simulink model "sampleModel7288_pp_1_1"  (R2018a)
settings: Solver=VariableStepAuto  StartTime=0.0  StopTime=10.0  RelTol=1e-3
undefined symbols (not defined in the file): DiscIntNeverNeededParam, sigbuilder_block
libraries: simulink x497
(part 1 of 10)
settings Model: Creator=cyfuzz  LastModifiedBy=shafiul
settings CodeAppCC: StateflowObjectComments=on

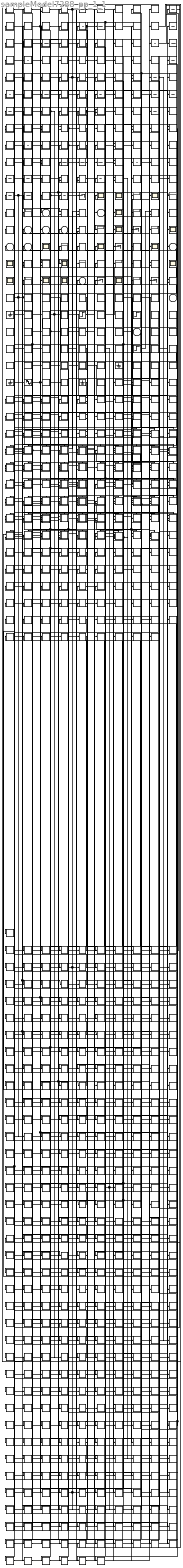
== system sampleModel7288_pp_1_1 ==
  cfblk180 : Inport
  cfblk198 : Inport  Port=2
  cfblk{1,9,50,54..55,58,83,85,88} (9 alike) : simulink/Discrete/Difference  ICPrevInput=0.0  OutMin=[]  OutMax=[]  OutDataTypeStr=double  OutputDataTypeScalingMode=double  OutDataType=fixdt(1, 16)  OutScaling=2^-10  DoSatur=off
  cfblk{10,20,40,56,59..60,102,106,111,114} (10 alike) : DiscreteIntegrator  OutDataTypeStr=double  ICPrevOutput=DiscIntNeverNeededParam  ICPrevScaledInput=DiscIntNeverNeededParam
  cfblk{28,77,89,100} (4 alike) : simulink/Discrete/Transfer Fcn Lead or Lag  PoleZ=0.95  ZeroZ=0.75  ICPrevOutput=0.0  ICPrevInput=0.0  DoSatur=off
      settings: SourceProductName=Simulink  SourceProductBaseCode=SL
  cfblk{5,16,49,53,61,69,96,101} (8 alike) : DiscreteTransferFcn  SampleTime=1
  cfblk{12,39,45,103} (4 alike) : simulink/Discrete/Transfer Fcn Real Zero  ZeroZ=0.75  ICPrevInput=0.0  DoSatur=off
      settings: SourceProductName=Simulink  SourceProductBaseCode=SL
  cfblk{71,80,92,97,104..105} (6 alike) : simulink/Continuous/PID Controller (2DOF)  Controller=PID  TimeDomain=Discrete-time  SampleTime=1  IntegratorMethod=Forward Euler  FilterMethod=Forward Euler  Form=Parallel  UseFilter=on  ControllerParametersSource=internal  P=1  I=1  D=0  N=100  b=1  c=1  InitialConditionSource=internal  InitialConditionForIntegrator=0  InitialConditionForFilter=0  ExternalReset=none  LimitOutput=off  UpperSaturationLimit=inf  LowerSaturationLimit=-inf  LinearizeAsGain=off  AntiWindupMode=none  Kb=1  TrackingMode=off  Kt=1  PParamMin=[]  PParamMax=[]  IParamMin=[]  IParamMax=[]  DParamMin=[]  DParamMax=[]  NParamMin=[]  NParamMax=[]  bParamMin=[]  bParamMax=[]  cParamMin=[]  cParamMax=[]  KbParamMin=[]  KbParamMax=[]  KtParamMin=[]  KtParamMax=[]  POutMin=[]  POutMax=[]  IOutMin=[]  IOutMax=[]  DOutMin=[]  DOutMax=[]  NOutMin=[]  NOutMax=[]  bOutMin=[]  bOutMax=[]  cOutMin=[]  cOutMax=[]  KbOutMin=[]  KbOutMax=[]  KtOutMin=[]  KtOutMax=[]  IntegratorOutMin=[]  IntegratorOutMax=[]  FilterOutMin=[]  FilterOutMax=[]  SumOutMin=[]  SumOutMax=[]  Sum1OutMin=[]  Sum1OutMax=[]  Sum2OutMin=[]  Sum2OutMax=[]  Sum3OutMin=[]  Sum3OutMax=[]  SumI1OutMin=[]  SumI1OutMax=[]  SumI2OutMin=[]  SumI2OutMax=[]  SumI3OutMin=[]  SumI3OutMax=[]  SumDOutMin=[]  SumDOutMax=[]  SaturationOutMin=[]  SaturationOutMax=[]  IntegratorContinuousStateAttributes=''  IntegratorStateMustResolveToSignalObject=off  IntegratorRTWStateStorageClass=Auto  FilterContinuousStateAttributes=''  FilterStateMustResolveToSignalObject=off  FilterRTWStateStorageClass=Auto  DifferentiatorICPrevScaledInput=0  DifferentiatorOutMin=[]  DifferentiatorOutMax=[]  FilterDiffOutCoefMin=[]  FilterDiffOutCoefMax=[]  SumDenOutMin=[]  SumDenOutMax=[]  SumNumOutMin=[]  SumNumOutMax=[]  ReciprocalOutMin=[]  ReciprocalOutMax=[]  DivideOutMin=[]  DivideOutMax=[]  TunerSelectOption=Transfer Function Based (PID Tuner App)
  cfblk{3,22,48,72..74,87,107} (8 alike) : Delay  DelayLengthSource=Input port  SampleTime=1
      settings: InputPortMap=u0,p1
  cfblk{43,65,76,84,91,108..109} (7 alike) : DiscreteZeroPole  Poles=[0 0.5]  Gain=1
  cfblk{7,11,44,52,63,90} (6 alike) : simulink/Discrete/Transfer Fcn First Order  PoleZ=0.95  ICPrevOutput=0.0  DoSatur=off
      settings: SourceProductName=Simulink
  cfblk{18,26,34..35,46,57,68,81,86,99,110} (11 alike) : simulink/Continuous/PID Controller  Controller=PID  TimeDomain=Discrete-time  SampleTime=1  IntegratorMethod=Forward Euler  FilterMethod=Forward Euler  Form=Parallel  UseFilter=on  ControllerParametersSource=internal  P=1  I=1  D=0  N=100  InitialConditionSource=internal  InitialConditionForIntegrator=0  InitialConditionForFilter=0  ExternalReset=none  LimitOutput=off  UpperSaturationLimit=inf  LowerSaturationLimit=-inf  LinearizeAsGain=off  AntiWindupMode=none  Kb=1  TrackingMode=off  Kt=1  PParamMin=[]  PParamMax=[]  IParamMin=[]  IParamMax=[]  DParamMin=[]  DParamMax=[]  NParamMin=[]  NParamMax=[]  KbParamMin=[]  KbParamMax=[]  KtParamMin=[]  KtParamMax=[]  POutMin=[]  POutMax=[]  IOutMin=[]  IOutMax=[]  DOutMin=[]  DOutMax=[]  NOutMin=[]  NOutMax=[]  KbOutMin=[]  KbOutMax=[]  KtOutMin=[]  KtOutMax=[]  IntegratorOutMin=[]  IntegratorOutMax=[]  FilterOutMin=[]  FilterOutMax=[]  SumOutMin=[]  SumOutMax=[]  SumI1OutMin=[]  SumI1OutMax=[]  SumI2OutMin=[]  SumI2OutMax=[]  SumI3OutMin=[]  SumI3OutMax=[]  SumDOutMin=[]  SumDOutMax=[]  SaturationOutMin=[]  SaturationOutMax=[]  IntegratorContinuousStateAttributes=''  IntegratorStateMustResolveToSignalObject=off  IntegratorRTWStateStorageClass=Auto  FilterContinuousStateAttributes=''  FilterStateMustResolveToSignalObject=off  FilterRTWStateStorageClass=Auto  DifferentiatorICPrevScaledInput=0  DifferentiatorOutMin=[]  DifferentiatorOutMax=[]  FilterDiffOutCoefMin=[]  FilterDiffOutCoefMax=[]  SumDenOutMin=[]  SumDenOutMax=[]  SumNumOutMin=[]  SumNumOutMax=[]  ReciprocalOutMin=[]  ReciprocalOutMax=[]  DivideOutMin=[]  DivideOutMax=[]  TunerSelectOption=Transfer Function Based (PID Tuner App)
  cfblk{6,23,30,94..95,112} (6 alike) : DiscreteFilter  SampleTime=1
  cfblk{8,19,24..25,31,37..38,62,64,67,113,320..375} (67 alike) : Delay  SampleTime=1
  cfblk{115,138,147,166,169} (5 alike) : Terminator
  cfblk{116..117,119,127,137,140,143,146,149,151,154,160..161,163..164,167} (16 alike) : Scope
      cfblk117 settings: Floating=on
      cfblk143 settings: Floating=on
      cfblk151 settings: Floating=on
      cfblk160 settings: Floating=on
      cfblk161 settings: Floating=on
      cfblk164 settings: Floating=on
      cfblk167 settings: Floating=on
  cfblk{118,120,122,128,136,139,144,155,157,162,168} (11 alike) : Display
  cfblk121 : ToWorkspace  VariableName=ajgaihg  SaveFormat=Timeseries  SampleTime=-1
  cfblk{124..125,129,135,152..153,159,170} (8 alike) : simulink/Sinks/XY Graph  xmin=-1  xmax=1  ymin=-1  ymax=1  st=-1
  cfblk{2,13..14,21,27,36,41..42,47,75} (10 alike) : simulink/Discrete/Tapped Delay  vinit=0.0  samptime=-1  NumDelays=1  DelayOrder=Oldest  includeCurrent=off
  cfblk130 : ToWorkspace  VariableName=uwfehsf  SaveFormat=Timeseries  SampleTime=-1
  cfblk131 : ToWorkspace  VariableName=zgsnsfd  SaveFormat=Timeseries  SampleTime=-1
  cfblk145 : ToWorkspace  VariableName=qxglayd  SaveFormat=Timeseries  SampleTime=-1
  cfblk148 : ToWorkspace  VariableName=ajdkbiq  SaveFormat=Timeseries  SampleTime=-1
  cfblk{15,29,32,51,82,98} (6 alike) : UnitDelay
  cfblk156 : ToWorkspace  VariableName=zvxkfyp  SaveFormat=Timeseries  SampleTime=-1
  cfblk158 : ToWorkspace  VariableName=xydmkth  SaveFormat=Timeseries  SampleTime=-1
  cfblk{4,17,33,70,79} (5 alike) : DiscreteStateSpace
  cfblk171 : simulink/Sources/Band-Limited White Noise  Cov=[0.1]  Ts=0.1  seed=[23341]
  cfblk{172,174,182,192,196,211,216} (7 alike) : simulink/Sources/Counter Limited  uplimit=7  tsamp=1
  cfblk173 : simulink/Sources/Band-Limited White Noise  Cov=[0.1]  Ts=0.1  seed=[23341]
  cfblk175 : DigitalClock
  cfblk176 : simulink/Sources/Counter Free-Running  NumBits=16  tsamp=1
  cfblk{177,179,191,197,204,207,226} (7 alike) : SignalGenerator  Units=rad/sec
  cfblk178 : simulink/Sources/Chirp Signal  f1=0.1  T=100  f2=1
  cfblk{181,217,221,225} (4 alike) : Ground
  cfblk183 : simulink/Sources/Ramp  slope=1  start=0  InitialOutput=0
  cfblk184 : simulink/Sources/Chirp Signal  f1=0.1  T=100  f2=1
  cfblk185 : Step  After=67  SampleTime=0
  cfblk{186,210,220,224} (4 alike) : simulink/Sources/Repeating Sequence  rep_seq_t=[0 2]  rep_seq_y=[0 2]
  cfblk{187,189..190,199,205,223} (6 alike) : DiscretePulseGenerator  PulseType=Time based  Period=10  PulseWidth=5
  cfblk188 : Step  After=98  SampleTime=0
  cfblk{193,206,212,219} (4 alike) : simulink/Sources/Repeating Sequence Interpolated  OutValues=[3 1 4 2 1].'  TimeValues=[0 0.1 0.5 0.6 1].'  LookUpMeth=Interpolation-Use End Values  tsamp=0.01  OutMin=[]  OutMax=[]  OutDataTypeStr=double  OutputDataTypeScalingMode=double  OutDataType=fixdt(0,8)  OutScaling=2^-10
  cfblk194 : UniformRandomNumber  SampleTime=0.1
  cfblk195 : UniformRandomNumber  SampleTime=0.1
  cfblk200 : Subsystem  Tag=STV Subsys  LoadFcn=sigbuilder_block('load');  StartFcn=sigbuilder_block('start');  StopFcn=sigbuilder_block('stop');  ClipboardFcn=sigbuilder_block('clipboard');  mask(Sigbuilder block){tuvar=[0:10]}
      mask help: Simulink:masks:SigbuilderBlock_MD
      mask init:
      | if ~strcmp(get_param(bdroot(gcbh),'SimulationStatus'),'stopped') tuvar = sigbuilder_block('maskInit'); end
      settings: CopyFcn=sigbuilder_block('copy');  DeleteFcn=sigbuilder_block('delete');  ModelCloseFcn=sigbuilder_block('modelClose');  PreSaveFcn=sigbuilder_block('preSave');  PauseFcn=sigbuilder_block('pause');  ContinueFcn=sigbuilder_block('continue');  NameChangeFcn=sigbuilder_block('namechange');  OpenFcn=sigbuilder_block('open',[437.6 199.2 550.4 400 ]);  CloseFcn=sigbuilder_block('close');
      mask Display: plot(0, 0, 100, 100,[2, 2, 32, 32, 2], [68, 8, 8, 68, 68],[32, 2], [38, 38], [32, 19, 2],[53, 60, 44], [32, 17, 17, 2],[16, 16, 31, 31]);txt = getActiveGroup(gcbh);text(2, 100, txt,'verticalAlignment', 'top');
  cfblk201 : simulink/Sources/Ramp  slope=1  start=0  InitialOutput=0
  cfblk202 : simulink/Sources/Repeating Sequence Stair  OutValues=[3 1 4 2 1].'  tsamp=1  OutMin=[]  OutMax=[]  OutDataTypeStr=double  OutputDataTypeScalingMode=double  OutDataType=fixdt(0,8)  ConRadixGroup=Best Precision: Vector-wise  OutScaling=2^-12
  cfblk203 : simulink/Sources/Repeating Sequence Stair  OutValues=[3 1 4 2 1].'  tsamp=1  OutMin=[]  OutMax=[]  OutDataTypeStr=double  OutputDataTypeScalingMode=double  OutDataType=fixdt(0,8)  ConRadixGroup=Best Precision: Vector-wise  OutScaling=2^-12
  cfblk208 : Step  After=14  SampleTime=0
  cfblk209 : simulink/Sources/Band-Limited White Noise  Cov=[0.1]  Ts=0.1  seed=[23341]
  cfblk213 : RandomNumber  SampleTime=0.1
  cfblk214 : Subsystem  Tag=STV Subsys  LoadFcn=sigbuilder_block('load');  StartFcn=sigbuilder_block('start');  StopFcn=sigbuilder_block('stop');  ClipboardFcn=sigbuilder_block('clipboard');  mask(Sigbuilder block){tuvar=[0:10]}
      mask help: Simulink:masks:SigbuilderBlock_MD
      mask init:
      | if ~strcmp(get_param(bdroot(gcbh),'SimulationStatus'),'stopped') tuvar = sigbuilder_block('maskInit'); end
      settings: CopyFcn=sigbuilder_block('copy');  DeleteFcn=sigbuilder_block('delete');  ModelCloseFcn=sigbuilder_block('modelClose');  PreSaveFcn=sigbuilder_block('preSave');  PauseFcn=sigbuilder_block('pause');  ContinueFcn=sigbuilder_block('continue');  NameChangeFcn=sigbuilder_block('namechange');  OpenFcn=sigbuilder_block('open',[437.6 199.2 550.4 400 ]);  CloseFcn=sigbuilder_block('close');
      mask Display: plot(0, 0, 100, 100,[2, 2, 32, 32, 2], [68, 8, 8, 68, 68],[32, 2], [38, 38], [32, 19, 2],[53, 60, 44], [32, 17, 17, 2],[16, 16, 31, 31]);txt = getActiveGroup(gcbh);text(2, 100, txt,'verticalAlignment', 'top');
  cfblk215 : Subsystem  Tag=STV Subsys  LoadFcn=sigbuilder_block('load');  StartFcn=sigbuilder_block('start');  StopFcn=sigbuilder_block('stop');  ClipboardFcn=sigbuilder_block('clipboard');  mask(Sigbuilder block){tuvar=[0:10]}
      mask help: Simulink:masks:SigbuilderBlock_MD
      mask init:
      | if ~strcmp(get_param(bdroot(gcbh),'SimulationStatus'),'stopped') tuvar = sigbuilder_block('maskInit'); end
      settings: CopyFcn=sigbuilder_block('copy');  DeleteFcn=sigbuilder_block('delete');  ModelCloseFcn=sigbuilder_block('modelClose');  PreSaveFcn=sigbuilder_block('preSave');  PauseFcn=sigbuilder_block('pause');  ContinueFcn=sigbuilder_block('continue');  NameChangeFcn=sigbuilder_block('namechange');  OpenFcn=sigbuilder_block('open',[437.6 199.2 550.4 400 ]);  CloseFcn=sigbuilder_block('close');
      mask Display: plot(0, 0, 100, 100,[2, 2, 32, 32, 2], [68, 8, 8, 68, 68],[32, 2], [38, 38], [32, 19, 2],[53, 60, 44], [32, 17, 17, 2],[16, 16, 31, 31]);txt = getActiveGroup(gcbh);text(2, 100, txt,'verticalAlignment', 'top');
  cfblk218 : simulink/Sources/Counter Free-Running  NumBits=16  tsamp=1
  cfblk222 : Sin  SampleTime=0
  cfblk{227..257} (31 alike) : If  SampleTime=1
  cfblk258 : Subsystem  TreatAsAtomicUnit=on
  cfblk259 : Subsystem  TreatAsAtomicUnit=on
  cfblk260 : Subsystem  TreatAsAtomicUnit=on
  cfblk261 : Subsystem  TreatAsAtomicUnit=on
  cfblk262 : Subsystem  TreatAsAtomicUnit=on
  cfblk263 : Subsystem  TreatAsAtomicUnit=on
  cfblk264 : Subsystem  TreatAsAtomicUnit=on
  cfblk265 : Subsystem  TreatAsAtomicUnit=on
  cfblk266 : Subsystem  TreatAsAtomicUnit=on
  cfblk267 : Subsystem  TreatAsAtomicUnit=on
  cfblk268 : Subsystem  TreatAsAtomicUnit=on
  cfblk269 : Subsystem  TreatAsAtomicUnit=on
  cfblk270 : Subsystem  TreatAsAtomicUnit=on
  cfblk271 : Subsystem  TreatAsAtomicUnit=on
  cfblk272 : Subsystem  TreatAsAtomicUnit=on
  cfblk273 : Subsystem  TreatAsAtomicUnit=on
  cfblk274 : Subsystem  TreatAsAtomicUnit=on
  cfblk275 : Subsystem  TreatAsAtomicUnit=on
  cfblk276 : Subsystem  TreatAsAtomicUnit=on
  cfblk277 : Subsystem  TreatAsAtomicUnit=on
  cfblk278 : Subsystem  TreatAsAtomicUnit=on
  cfblk279 : Subsystem  TreatAsAtomicUnit=on
  cfblk280 : Subsystem  TreatAsAtomicUnit=on
  cfblk281 : Subsystem  TreatAsAtomicUnit=on
  cfblk282 : Subsystem  TreatAsAtomicUnit=on
  cfblk283 : Subsystem  TreatAsAtomicUnit=on
  cfblk284 : Subsystem  TreatAsAtomicUnit=on
  cfblk285 : Subsystem  TreatAsAtomicUnit=on
  cfblk286 : Subsystem  TreatAsAtomicUnit=on
  cfblk287 : Subsystem  TreatAsAtomicUnit=on
  cfblk288 : Subsystem  TreatAsAtomicUnit=on
  cfblk289 : Subsystem  TreatAsAtomicUnit=on
  cfblk290 : Subsystem  TreatAsAtomicUnit=on
  cfblk291 : Subsystem  TreatAsAtomicUnit=on
  cfblk292 : Subsystem  TreatAsAtomicUnit=on
  cfblk293 : Subsystem  TreatAsAtomicUnit=on
  cfblk294 : Subsystem  TreatAsAtomicUnit=on
  cfblk295 : Subsystem  TreatAsAtomicUnit=on
  cfblk296 : Subsystem  TreatAsAtomicUnit=on
  cfblk297 : Subsystem  TreatAsAtomicUnit=on
  cfblk298 : Subsystem  TreatAsAtomicUnit=on
  cfblk299 : Subsystem  TreatAsAtomicUnit=on
  cfblk300 : Subsystem  TreatAsAtomicUnit=on
  cfblk301 : Subsystem  TreatAsAtomicUnit=on
  cfblk302 : Subsystem  TreatAsAtomicUnit=on
  cfblk303 : Subsystem  TreatAsAtomicUnit=on
  cfblk304 : Subsystem  TreatAsAtomicUnit=on
  cfblk305 : Subsystem  TreatAsAtomicUnit=on
  cfblk306 : Subsystem  TreatAsAtomicUnit=on
  cfblk307 : Subsystem  TreatAsAtomicUnit=on
  cfblk308 : Subsystem  TreatAsAtomicUnit=on
  cfblk309 : Subsystem  TreatAsAtomicUnit=on
  cfblk310 : Subsystem  TreatAsAtomicUnit=on
  cfblk311 : Subsystem  TreatAsAtomicUnit=on
  cfblk312 : Subsystem  TreatAsAtomicUnit=on
  cfblk313 : Subsystem  TreatAsAtomicUnit=on
  cfblk314 : Subsystem  TreatAsAtomicUnit=on
  cfblk315 : Subsystem  TreatAsAtomicUnit=on
  cfblk316 : Subsystem  TreatAsAtomicUnit=on
  cfblk317 : Subsystem  TreatAsAtomicUnit=on
  cfblk318 : Subsystem  TreatAsAtomicUnit=on
  cfblk319 : Subsystem  TreatAsAtomicUnit=on
  cfblk{376..379} (4 alike) : DataTypeConversion  OutDataTypeStr=double
  cfblk66 : Delay  ShowEnablePort=on  SampleTime=1
      settings: InputPortMap=u0,e6
  cfblk78 : Delay  ShowEnablePort=on  SampleTime=1
      settings: InputPortMap=u0,e6
  cfblk93 : Delay  ShowEnablePort=on  SampleTime=1
      settings: InputPortMap=u0,e6
  cyemi_{0..4,6..11,13..66,68..75,117..119,168..169,215..216,231..232,270,284,300..301,330,334..336,352,413..414,430..435,444..447,457..458,465..466,474,476,519..520,540,550..552,560..562,628..630,634..635,677,683..685,695,723,763..764,777,790..792,805,840,848..850,862..863,879,891..893,928..930,936..938,967,1014..1016,1030..1033,1042..1044,1128..1131,1139..1140,1235,1244..1247,1259..1260,1269..1271,1293,1344..1345,1359,1369,1434..1437,1493..1494,1542,1592..1593,1639..1641,1669,1696..1697,1733..1738,1768..1769,1813..1817,1829..1891,1893,1895..1938,1940..1957,1959..1974} (354 alike) : DataTypeConversion  OutDataTypeStr=double
  cyemi_{5,12,475,559,935,1368,1892,1894,1939} (9 alike) : DataTypeConversion  OutDataTypeStr=uint8
  cyemi_1958 : DataTypeConversion  OutDataTypeStr=uint32
  cyemi_67 : DataTypeConversion  OutDataTypeStr=uint16
  cyemi_722 : DataTypeConversion  OutDataTypeStr=uint16
  cyemi_806 : DataTypeConversion  OutDataTypeStr=uint32
  cfblk123 : Outport
  cfblk126 : Outport  Port=2
  cfblk132 : Outport  Port=3
  cfblk133 : Outport  Port=4
  cfblk134 : Outport  Port=5
  cfblk141 : Outport  Port=6
  cfblk142 : Outport  Port=7
  cfblk150 : Outport  Port=8
  cfblk165 : Outport  Port=9
  wires:
  cfblk264/1(cfblk2) -> cfblk125/1
  cfblk287/2(cfblk13) -> cfblk119/1
  cfblk208/1 -> cfblk129/1
  cfblk193/1 -> cyemi_1593/1, cyemi_1957/1
  cfblk11/1 -> cfblk124/1
  cfblk63/1 -> cyemi_1849/1, cyemi_1852/1
  cfblk304/1(cfblk2) -> cfblk159/1
  cfblk213/1 -> cfblk159/2
  cfblk309/1(cfblk2) -> cfblk132/1
  cfblk180/1 -> cfblk144/1
  cfblk270/1(cfblk2) -> cfblk127/1
  cfblk206/1 -> cyemi_862/1, cyemi_1945/1
  cfblk86/1 -> cyemi_69/1, cyemi_1641/1
  cfblk107/1 -> cyemi_1270/1, cyemi_1866/1
  cfblk49/1 -> cfblk137/1, cyemi_1848/1
  cfblk301/1(cfblk2) -> cfblk163/1
  cfblk39/1 -> cyemi_414/1, cyemi_1815/1
  cfblk183/1 -> cfblk147/1, cyemi_929/1
  cfblk87/1 -> cyemi_21/1, cyemi_1878/1
  cfblk8/1 -> cfblk136/1, cyemi_1436/1
  cfblk15/1 -> cyemi_1033/1, cyemi_1840/1
  cfblk47/1 -> cfblk154/1
  cfblk222/1 -> cfblk133/1, cyemi_1905/1
  cfblk43/1 -> cyemi_270/1, cyemi_1946/1
  cfblk195/1 -> cfblk126/1
  cfblk64/1 -> cfblk138/1
  cfblk75/1 -> cfblk123/1
  cfblk186/1 -> cfblk128/1
  cfblk284/1(cfblk2) -> cfblk125/2
  cfblk288/1(cfblk2) -> cfblk118/1
  cfblk314/2(cfblk9) -> cfblk152/1
  cfblk93/1 -> cfblk152/2
  cfblk307/2(cfblk13) -> cyemi_628/1, cyemi_1865/1
  cfblk277/1(cfblk2) -> cfblk165/1, cyemi_118/1
  cfblk84/1 -> cfblk153/1, cyemi_433/1
  cfblk65/1 -> cyemi_474/1, cyemi_1890/1
  cfblk53/1 -> cfblk120/1, cyemi_1965/1
  cfblk18/1 -> cyemi_63/1, cyemi_1640/1
  cfblk98/1 -> cfblk129/2
  cfblk312/3(cfblk14) -> cyemi_520/1, cyemi_1845/1
  cfblk220/1 -> cfblk134/1
  cfblk306/1(cfblk2) -> cfblk116/1
  cfblk12/1 -> cfblk124/2, cyemi_1927/1
  cfblk199/1 -> cyemi_928/1, cyemi_936/1
  cfblk315/2(cfblk8) -> cyemi_562/1, cyemi_1901/1
  cfblk56/1 -> cfblk157/1
  cfblk284/3(cfblk13) -> cfblk169/1
  cfblk179/1 -> cfblk141/1
  cfblk269/2(cfblk15) -> cfblk150/1
  cfblk171/1 -> cfblk115/1, cyemi_683/1, cyemi_42/1
  cfblk306/2(cfblk9) -> cyemi_2/1, cyemi_1842/1
  cfblk113/1 -> cyemi_1895/1, cyemi_1951/1
  cfblk51/1 -> cyemi_56/1, cyemi_434/1
  cfblk4/1 -> cyemi_1933/1, cyemi_1943/1, cyemi_684/1
  cfblk298/4(cfblk15) -> cfblk170/1, cfblk142/1
  cfblk44/1 -> cyemi_15/1, cyemi_630/1, cyemi_1817/1
  cfblk192/1 -> cfblk155/1
  cfblk268/1(cfblk2) -> cfblk162/1
  cfblk22/1 -> cfblk168/1
  cfblk37/1 -> cfblk153/2
  cfblk67/1 -> cyemi_685/1, cyemi_1909/1
  cfblk300/1(cfblk2) -> cfblk166/1
  cfblk262/1(cfblk2) -> cyemi_11/1, cyemi_1867/1
  cfblk278/1(cfblk2) -> cfblk122/1
  cfblk80/1 -> cyemi_1898/1, cyemi_1928/1
  cfblk288/4(cfblk14) -> cyemi_930/1, cyemi_1854/1, cyemi_848/1
  cfblk41/1 -> cfblk140/1
  cfblk272/2(cfblk8) -> cyemi_39/1, cyemi_1863/1
  cfblk305/3(cfblk12) -> cyemi_1846/1, cyemi_1967/1
  cfblk204/1 -> cfblk135/1
  cfblk279/3(cfblk9) -> cyemi_1843/1, cyemi_1844/1
  cfblk111/1 -> cyemi_24/1, cyemi_1922/1, cyemi_476/1
  cfblk196/1 -> cyemi_12/1, cyemi_475/1
  cfblk317/2(cfblk17) -> cfblk146/1, cyemi_1916/1, cyemi_1900/1
  cfblk261/1(cfblk2) -> cfblk149/1
  cfblk308/2(cfblk10) -> cyemi_33/1, cyemi_1880/1
  cfblk259/4(cfblk16) -> cyemi_1838/1, cyemi_1839/1
  cfblk271/3(cfblk15) -> cfblk170/2
  cfblk74/1 -> cyemi_119/1, cyemi_1829/1
  cfblk311/4(cfblk17) -> cfblk135/2
  cfblk283/2(cfblk7) -> cfblk139/1
  cfblk227/1 -> cfblk258/Action
  cfblk227/2 -> cfblk259/Action
  cfblk228/1 -> cfblk260/Action
  cfblk228/2 -> cfblk261/Action
  cfblk229/1 -> cfblk262/Action
  cfblk229/2 -> cfblk263/Action
  cfblk230/1 -> cfblk264/Action
  cfblk230/2 -> cfblk265/Action
  cfblk231/1 -> cfblk266/Action
  cfblk231/2 -> cfblk267/Action
  cfblk232/1 -> cfblk268/Action
  cfblk232/2 -> cfblk269/Action
  cfblk233/1 -> cfblk270/Action
  cfblk233/2 -> cfblk271/Action
  cfblk234/1 -> cfblk272/Action
  cfblk234/2 -> cfblk273/Action
  cfblk235/1 -> cfblk274/Action
  cfblk235/2 -> cfblk275/Action
  cfblk236/1 -> cfblk276/Action
  cfblk236/2 -> cfblk277/Action
  cfblk237/1 -> cfblk278/Action
  cfblk237/2 -> cfblk279/Action
  cfblk238/1 -> cfblk280/Action
  cfblk238/2 -> cfblk281/Action
  cfblk239/1 -> cfblk282/Action
  cfblk239/2 -> cfblk283/Action
  cfblk240/1 -> cfblk284/Action
  cfblk240/2 -> cfblk285/Action
  cfblk241/1 -> cfblk286/Action
  cfblk241/2 -> cfblk287/Action
  cfblk242/1 -> cfblk288/Action
  cfblk242/2 -> cfblk289/Action
  cfblk243/1 -> cfblk290/Action
  cfblk243/2 -> cfblk291/Action
  cfblk244/1 -> cfblk292/Action
  cfblk244/2 -> cfblk293/Action
  cfblk245/1 -> cfblk294/Action
  cfblk245/2 -> cfblk295/Action
  cfblk246/1 -> cfblk296/Action
  cfblk246/2 -> cfblk297/Action
  cfblk247/1 -> cfblk298/Action
  cfblk247/2 -> cfblk299/Action
  cfblk248/1 -> cfblk300/Action
  cfblk248/2 -> cfblk301/Action
  cfblk249/1 -> cfblk302/Action
  cfblk249/2 -> cfblk303/Action
  cfblk250/1 -> cfblk304/Action
  cfblk250/2 -> cfblk305/Action
  cfblk251/1 -> cfblk306/Action
  cfblk251/2 -> cfblk307/Action
  cfblk252/1 -> cfblk308/Action
  cfblk252/2 -> cfblk309/Action
  cfblk253/1 -> cfblk310/Action
  cfblk253/2 -> cfblk311/Action
  cfblk254/1 -> cfblk312/Action
  cfblk254/2 -> cfblk313/Action
  cfblk255/1 -> cfblk314/Action
  cfblk255/2 -> cfblk315/Action
  cfblk256/1 -> cfblk316/Action
  cfblk256/2 -> cfblk317/Action
  cfblk257/1 -> cfblk318/Action
  cfblk257/2 -> cfblk319/Action
  cyemi_0/1 -> cfblk1/1
  cfblk336/1 -> cyemi_0/1
  cyemi_1/1 -> cfblk10/1
  cfblk210/1 -> cyemi_1/1
  cyemi_2/1 -> cfblk100/1
  cyemi_3/1 -> cfblk101/1
  cfblk25/1 -> cyemi_3/1
  cyemi_4/1 -> cfblk102/1
  cfblk305/1(cfblk2) -> cyemi_4/1
  cyemi_5/1 -> cfblk103/1
  cfblk182/1 -> cyemi_5/1
  cyemi_6/1 -> cfblk104/1
  cfblk280/2(cfblk13) -> cyemi_6/1
  cyemi_7/1 -> cfblk104/2
  cfblk295/2(cfblk9) -> cyemi_7/1
  cyemi_8/1 -> cfblk105/1
  cfblk312/2(cfblk13) -> cyemi_8/1
  cyemi_9/1 -> cfblk105/2
  cfblk58/1 -> cyemi_9/1
  cyemi_10/1 -> cfblk106/1
  cfblk35/1 -> cyemi_10/1
  cyemi_11/1 -> cfblk107/1
  cyemi_12/1 -> cfblk107/2
  cyemi_13/1 -> cfblk108/1
  cfblk59/1 -> cyemi_13/1
  cyemi_14/1 -> cfblk109/1
  cfblk271/1(cfblk2) -> cyemi_14/1
  cyemi_15/1 -> cfblk11/1
  cyemi_16/1 -> cfblk110/1
  cfblk377/1 -> cyemi_16/1
  cyemi_17/1 -> cfblk111/1
  cfblk293/1(cfblk2) -> cyemi_17/1
  cyemi_18/1 -> cfblk112/1
  cfblk108/1 -> cyemi_18/1
  cyemi_19/1 -> cfblk113/1
  cfblk265/1(cfblk2) -> cyemi_19/1
  cyemi_20/1 -> cfblk114/1
  cfblk311/3(cfblk16) -> cyemi_20/1
  cyemi_21/1 -> cfblk12/1
  cyemi_22/1 -> cfblk121/1
  cfblk292/1(cfblk2) -> cyemi_22/1
  cyemi_23/1 -> cfblk13/1
  cfblk77/1 -> cyemi_23/1
  cyemi_24/1 -> cfblk130/1
  cyemi_25/1 -> cfblk131/1
  cfblk94/1 -> cyemi_25/1
  cyemi_26/1 -> cfblk14/1
  cfblk221/1 -> cyemi_26/1
  cyemi_27/1 -> cfblk145/1
  cfblk280/1(cfblk2) -> cyemi_27/1
  cyemi_28/1 -> cfblk148/1
  cfblk274/1(cfblk2) -> cyemi_28/1
  cyemi_29/1 -> cfblk15/1
  cfblk177/1 -> cyemi_29/1
  cyemi_30/1 -> cfblk156/1
  cfblk215/1(Signal 1) -> cyemi_30/1
  cyemi_31/1 -> cfblk158/1
  cfblk266/2(cfblk6) -> cyemi_31/1
  cyemi_32/1 -> cfblk16/1
  cfblk68/1 -> cyemi_32/1
  cyemi_33/1 -> cfblk17/1
  cyemi_34/1 -> cfblk18/1
  cfblk226/1 -> cyemi_34/1
  cyemi_35/1 -> cfblk19/1
  cfblk319/1(cfblk2) -> cyemi_35/1
  cyemi_36/1 -> cfblk2/1
  cfblk24/1 -> cyemi_36/1
  cyemi_37/1 -> cfblk20/1
  cfblk290/1(cfblk2) -> cyemi_37/1
  cyemi_38/1 -> cfblk21/1
  cfblk275/1(cfblk2) -> cyemi_38/1
  cyemi_39/1 -> cfblk22/1
  cyemi_40/1 -> cfblk22/2
  cfblk178/1 -> cyemi_40/1
  cyemi_41/1 -> cfblk227/1
  cfblk191/1 -> cyemi_41/1
  cyemi_42/1 -> cfblk228/1
  cyemi_43/1 -> cfblk229/1
  cfblk375/1 -> cyemi_43/1
  cyemi_44/1 -> cfblk23/1
  cfblk38/1 -> cyemi_44/1
  cyemi_45/1 -> cfblk230/1
  cfblk374/1 -> cyemi_45/1
  cyemi_46/1 -> cfblk231/1
  cfblk346/1 -> cyemi_46/1
  cyemi_47/1 -> cfblk232/1
  cfblk370/1 -> cyemi_47/1
  cyemi_48/1 -> cfblk233/1
  cfblk367/1 -> cyemi_48/1
  cyemi_49/1 -> cfblk234/1
  cfblk355/1 -> cyemi_49/1
  cyemi_50/1 -> cfblk235/1
  cfblk269/3(cfblk16) -> cyemi_50/1
  cyemi_51/1 -> cfblk236/1
  cfblk279/1(cfblk2) -> cyemi_51/1
  cyemi_52/1 -> cfblk237/1
  cfblk332/1 -> cyemi_52/1
  cyemi_53/1 -> cfblk238/1
  cfblk92/1 -> cyemi_53/1
  cyemi_54/1 -> cfblk239/1
  cfblk308/1(cfblk2) -> cyemi_54/1
  cyemi_55/1 -> cfblk24/1
  cfblk292/3(cfblk13) -> cyemi_55/1
  cyemi_56/1 -> cfblk240/1
  cyemi_57/1 -> cfblk241/1
  cfblk267/1(cfblk2) -> cyemi_57/1
  cyemi_58/1 -> cfblk242/1
  cfblk201/1 -> cyemi_58/1
  cyemi_59/1 -> cfblk243/1
  cfblk30/1 -> cyemi_59/1
  cyemi_60/1 -> cfblk244/1
  cfblk46/1 -> cyemi_60/1
  cyemi_61/1 -> cfblk245/1
  cfblk55/1 -> cyemi_61/1
  cyemi_62/1 -> cfblk246/1
  cfblk318/1(cfblk2) -> cyemi_62/1
  cyemi_63/1 -> cfblk247/1
  cyemi_64/1 -> cfblk248/1
  cfblk175/1 -> cyemi_64/1
  cyemi_65/1 -> cfblk249/1
  cfblk357/1 -> cyemi_65/1
  cyemi_66/1 -> cfblk25/1
  cfblk286/2(cfblk8) -> cyemi_66/1
  cyemi_67/1 -> cfblk250/1
  cfblk218/1 -> cyemi_67/1
  cyemi_68/1 -> cfblk251/1
  cfblk298/3(cfblk14) -> cyemi_68/1
  cyemi_69/1 -> cfblk252/1
  cyemi_70/1 -> cfblk253/1
  cfblk13/1 -> cyemi_70/1
  cyemi_71/1 -> cfblk254/1
  cfblk198/1 -> cyemi_71/1
  cyemi_72/1 -> cfblk255/1
  cfblk369/1 -> cyemi_72/1
  cyemi_73/1 -> cfblk256/1
  cfblk78/1 -> cyemi_73/1
  cyemi_74/1 -> cfblk257/1
  cfblk79/1 -> cyemi_74/1
  cyemi_75/1 -> cfblk258/1(cfblk1)
  cfblk266/1(cfblk2) -> cyemi_75/1
  cyemi_117/1 -> cfblk259/1(cfblk1)
  cfblk266/3(cfblk7) -> cyemi_117/1
  cyemi_118/1 -> cfblk259/2(cfblk12)
  cyemi_119/1 -> cfblk259/3(cfblk13)
  cyemi_168/1 -> cfblk26/1
  cfblk276/1(cfblk2) -> cyemi_168/1
  cyemi_169/1 -> cfblk260/1(cfblk1)
  cfblk181/1 -> cyemi_169/1
  cyemi_215/1 -> cfblk261/1(cfblk1)
  cfblk224/1 -> cyemi_215/1
  cyemi_216/1 -> cfblk261/2(cfblk12)
  cfblk42/1 -> cyemi_216/1
  cyemi_231/1 -> cfblk262/1(cfblk1)
  cfblk343/1 -> cyemi_231/1
  cyemi_232/1 -> cfblk262/2(cfblk7)
  cfblk7/1 -> cyemi_232/1
  cyemi_270/1 -> cfblk263/1(cfblk1)
  cyemi_284/1 -> cfblk264/1(cfblk1)
  cfblk185/1 -> cyemi_284/1
  cyemi_300/1 -> cfblk265/1(cfblk1)
  cfblk194/1 -> cyemi_300/1
  cyemi_301/1 -> cfblk265/2(cfblk8)
  cfblk303/1(cfblk2) -> cyemi_301/1
  cyemi_330/1 -> cfblk266/1(cfblk1)
  cfblk372/1 -> cyemi_330/1
  cyemi_334/1 -> cfblk267/1(cfblk1)
  cfblk361/1 -> cyemi_334/1
  cyemi_335/1 -> cfblk267/2(cfblk15)
  cfblk365/1 -> cyemi_335/1
  cyemi_336/1 -> cfblk267/3(cfblk16)
  cfblk299/1(cfblk2) -> cyemi_336/1
  cyemi_352/1 -> cfblk268/1(cfblk1)
  cfblk207/1 -> cyemi_352/1
  cyemi_413/1 -> cfblk269/1(cfblk1)
  cfblk32/1 -> cyemi_413/1
  cyemi_414/1 -> cfblk269/2(cfblk14)
  cyemi_430/1 -> cfblk27/1
  cfblk71/1 -> cyemi_430/1
  cyemi_431/1 -> cfblk270/1(cfblk1)
  cfblk81/1 -> cyemi_431/1
  cyemi_432/1 -> cfblk270/2(cfblk10)
  cfblk352/1 -> cyemi_432/1
  cyemi_433/1 -> cfblk270/3(cfblk11)
  cyemi_434/1 -> cfblk270/4(cfblk12)
  cyemi_435/1 -> cfblk270/5(cfblk13)
  cfblk329/1 -> cyemi_435/1
  cyemi_444/1 -> cfblk271/1(cfblk1)
  cfblk349/1 -> cyemi_444/1
  cyemi_445/1 -> cfblk271/2(cfblk11)
  cfblk344/1 -> cyemi_445/1
  cyemi_446/1 -> cfblk271/3(cfblk12)
  cfblk188/1 -> cyemi_446/1
  cyemi_447/1 -> cfblk271/4(cfblk13)
  cfblk350/1 -> cyemi_447/1
  cyemi_457/1 -> cfblk272/1(cfblk1)
  cfblk348/1 -> cyemi_457/1
  cyemi_458/1 -> cfblk272/2(cfblk7)
  cfblk28/1 -> cyemi_458/1
  cyemi_465/1 -> cfblk273/1(cfblk1)
  cfblk270/2(cfblk14) -> cyemi_465/1
  cyemi_466/1 -> cfblk273/2(cfblk10)
  cfblk373/1 -> cyemi_466/1
  cyemi_474/1 -> cfblk274/1(cfblk1)
  cyemi_475/1 -> cfblk274/2(cfblk11)
  cyemi_476/1 -> cfblk274/3(cfblk12)
  cyemi_519/1 -> cfblk275/1(cfblk1)
  cfblk48/1 -> cyemi_519/1
  cyemi_520/1 -> cfblk275/2(cfblk16)
  cyemi_540/1 -> cfblk276/1(cfblk1)
  cfblk289/1(cfblk2) -> cyemi_540/1
  cyemi_550/1 -> cfblk277/1(cfblk1)
  cfblk323/1 -> cyemi_550/1
  cyemi_551/1 -> cfblk277/2(cfblk8)
  cfblk62/1 -> cyemi_551/1
  cyemi_552/1 -> cfblk277/3(cfblk9)
  cfblk265/2(cfblk9) -> cyemi_552/1
  cyemi_559/1 -> cfblk278/1(cfblk1)
  cfblk309/2(cfblk12) -> cyemi_559/1
  cyemi_560/1 -> cfblk278/2(cfblk14)
  cfblk16/1 -> cyemi_560/1
  cyemi_561/1 -> cfblk278/3(cfblk15)
  cfblk328/1 -> cyemi_561/1
  cyemi_562/1 -> cfblk278/4(cfblk16)
  cyemi_628/1 -> cfblk279/1(cfblk1)
  cyemi_629/1 -> cfblk279/2(cfblk6)
  cfblk290/2(cfblk13) -> cyemi_629/1
  cyemi_630/1 -> cfblk279/3(cfblk7)
  cyemi_634/1 -> cfblk28/1
  cfblk260/1(cfblk2) -> cyemi_634/1
  cyemi_635/1 -> cfblk280/1(cfblk1)
  cfblk316/1(cfblk2) -> cyemi_635/1
  cyemi_677/1 -> cfblk281/1(cfblk1)
  cfblk184/1 -> cyemi_677/1
  cyemi_683/1 -> cfblk282/1(cfblk1)
  cyemi_684/1 -> cfblk282/2(cfblk9)
  cyemi_685/1 -> cfblk282/3(cfblk10)
  cyemi_695/1 -> cfblk283/1(cfblk1)
  cfblk362/1 -> cyemi_695/1
  cyemi_722/1 -> cfblk284/1(cfblk1)
  cfblk176/1 -> cyemi_722/1
  cyemi_723/1 -> cfblk284/2(cfblk11)
  cfblk274/2(cfblk13) -> cyemi_723/1
  cyemi_763/1 -> cfblk285/1(cfblk1)
  cfblk83/1 -> cyemi_763/1
  cyemi_764/1 -> cfblk285/2(cfblk12)
  cfblk114/1 -> cyemi_764/1
  cyemi_777/1 -> cfblk286/1(cfblk1)
  cfblk331/1 -> cyemi_777/1
  cyemi_790/1 -> cfblk287/1(cfblk1)
  cfblk321/1 -> cyemi_790/1
  cyemi_791/1 -> cfblk287/2(cfblk11)
  cfblk356/1 -> cyemi_791/1
  cyemi_792/1 -> cfblk287/3(cfblk12)
  cfblk345/1 -> cyemi_792/1
  cyemi_805/1 -> cfblk288/1(cfblk1)
  cfblk285/1(cfblk2) -> cyemi_805/1
  cyemi_806/1 -> cfblk288/2(cfblk11)
  cfblk311/1(cfblk2) -> cyemi_806/1
  cyemi_840/1 -> cfblk289/1(cfblk1)
  cfblk313/1(cfblk2) -> cyemi_840/1
  cyemi_848/1 -> cfblk29/1
  cyemi_849/1 -> cfblk290/1(cfblk1)
  cfblk312/1(cfblk2) -> cyemi_849/1
  cyemi_850/1 -> cfblk290/2(cfblk12)
  cfblk264/3(cfblk15) -> cyemi_850/1
  cyemi_862/1 -> cfblk291/1(cfblk1)
  cyemi_863/1 -> cfblk291/2(cfblk11)
  cfblk52/1 -> cyemi_863/1
  cyemi_879/1 -> cfblk292/1(cfblk1)
  cfblk316/2(cfblk9) -> cyemi_879/1
  cyemi_891/1 -> cfblk293/1(cfblk1)
  cfblk324/1 -> cyemi_891/1
  cyemi_892/1 -> cfblk293/2(cfblk9)
  cfblk327/1 -> cyemi_892/1
  cyemi_893/1 -> cfblk293/3(cfblk10)
  cfblk258/1(cfblk2) -> cyemi_893/1
  cyemi_928/1 -> cfblk294/1(cfblk1)
  cyemi_929/1 -> cfblk294/2(cfblk7)
  cyemi_930/1 -> cfblk294/3(cfblk8)
  cyemi_935/1 -> cfblk295/1(cfblk1)
  cfblk103/1 -> cyemi_935/1
  cyemi_936/1 -> cfblk295/2(cfblk6)
  cyemi_937/1 -> cfblk295/3(cfblk7)
  cfblk99/1 -> cyemi_937/1
  cyemi_938/1 -> cfblk295/4(cfblk8)
  cfblk265/4(cfblk11) -> cyemi_938/1
  cyemi_967/1 -> cfblk296/1(cfblk1)
  cfblk360/1 -> cyemi_967/1
  cyemi_1014/1 -> cfblk297/1(cfblk1)
  cfblk89/1 -> cyemi_1014/1
  cyemi_1015/1 -> cfblk297/2(cfblk10)
  cfblk342/1 -> cyemi_1015/1
  cyemi_1016/1 -> cfblk297/3(cfblk11)
  cfblk340/1 -> cyemi_1016/1
  cyemi_1030/1 -> cfblk298/1(cfblk1)
  cfblk270/3(cfblk15) -> cyemi_1030/1
  cyemi_1031/1 -> cfblk298/2(cfblk10)
  cfblk335/1 -> cyemi_1031/1
  cyemi_1032/1 -> cfblk298/3(cfblk11)
  cfblk353/1 -> cyemi_1032/1
  cyemi_1033/1 -> cfblk298/4(cfblk12)
  cyemi_1042/1 -> cfblk299/1(cfblk1)
  cfblk330/1 -> cyemi_1042/1
  cyemi_1043/1 -> cfblk299/2(cfblk13)
  cfblk60/1 -> cyemi_1043/1
  cyemi_1044/1 -> cfblk299/3(cfblk14)
  cfblk368/1 -> cyemi_1044/1
  cyemi_1128/1 -> cfblk3/1
  cfblk10/1 -> cyemi_1128/1
  cyemi_1129/1 -> cfblk3/2
  cfblk259/3(cfblk15) -> cyemi_1129/1
  cyemi_1130/1 -> cfblk30/1
  cfblk31/1 -> cyemi_1130/1
  cyemi_1131/1 -> cfblk300/1(cfblk1)
  cfblk85/1 -> cyemi_1131/1
  cyemi_1139/1 -> cfblk301/1(cfblk1)
  cfblk260/3(cfblk16) -> cyemi_1139/1
  cyemi_1140/1 -> cfblk301/2(cfblk15)
  cfblk268/2(cfblk10) -> cyemi_1140/1
  cyemi_1235/1 -> cfblk302/1(cfblk1)
  cfblk359/1 -> cyemi_1235/1
  cyemi_1244/1 -> cfblk303/1(cfblk1)
  cfblk1/1 -> cyemi_1244/1
  cyemi_1245/1 -> cfblk303/2(cfblk13)
  cfblk371/1 -> cyemi_1245/1
  cyemi_1246/1 -> cfblk303/3(cfblk14)
  cfblk341/1 -> cyemi_1246/1
  cyemi_1247/1 -> cfblk303/4(cfblk15)
  cfblk325/1 -> cyemi_1247/1
  cyemi_1259/1 -> cfblk304/1(cfblk1)
  cfblk112/1 -> cyemi_1259/1
  cyemi_1260/1 -> cfblk304/2(cfblk8)
  cfblk283/1(cfblk2) -> cyemi_1260/1
  cyemi_1269/1 -> cfblk305/1(cfblk1)
  cfblk351/1 -> cyemi_1269/1
  cyemi_1270/1 -> cfblk305/2(cfblk9)
  cyemi_1271/1 -> cfblk305/3(cfblk10)
  cfblk326/1 -> cyemi_1271/1
  cyemi_1293/1 -> cfblk306/1(cfblk1)
  cfblk90/1 -> cyemi_1293/1
  cyemi_1344/1 -> cfblk307/1(cfblk1)
  cfblk197/1 -> cyemi_1344/1
  cyemi_1345/1 -> cfblk307/2(cfblk12)
  cfblk45/1 -> cyemi_1345/1
  cyemi_1359/1 -> cfblk308/1(cfblk1)
  cfblk96/1 -> cyemi_1359/1
  cyemi_1368/1 -> cfblk309/1(cfblk1)
  cfblk172/1 -> cyemi_1368/1
  cyemi_1369/1 -> cfblk309/2(cfblk11)
  cfblk376/1 -> cyemi_1369/1
  cyemi_1434/1 -> cfblk31/1
  cfblk282/1(cfblk2) -> cyemi_1434/1
  cyemi_1435/1 -> cfblk310/1(cfblk1)
  cfblk212/1 -> cyemi_1435/1
  cyemi_1436/1 -> cfblk310/2(cfblk14)
  cyemi_1437/1 -> cfblk310/3(cfblk15)
  cfblk333/1 -> cyemi_1437/1
  cyemi_1493/1 -> cfblk311/1(cfblk1)
  cfblk364/1 -> cyemi_1493/1
  cyemi_1494/1 -> cfblk311/2(cfblk14)
  cfblk337/1 -> cyemi_1494/1
  cyemi_1542/1 -> cfblk312/1(cfblk1)
  cfblk292/2(cfblk12) -> cyemi_1542/1
  cyemi_1592/1 -> cfblk313/1(cfblk1)
  cfblk303/2(cfblk16) -> cyemi_1592/1
  cyemi_1593/1 -> cfblk313/2(cfblk13)
  cyemi_1639/1 -> cfblk314/1(cfblk1)
  cfblk347/1 -> cyemi_1639/1
  cyemi_1640/1 -> cfblk314/2(cfblk7)
  cyemi_1641/1 -> cfblk314/3(cfblk8)
  cyemi_1669/1 -> cfblk315/1(cfblk1)
  cfblk34/1 -> cyemi_1669/1
  cyemi_1696/1 -> cfblk316/1(cfblk1)
  cfblk338/1 -> cyemi_1696/1
  cyemi_1697/1 -> cfblk316/2(cfblk8)
  cfblk339/1 -> cyemi_1697/1
  cyemi_1733/1 -> cfblk317/1(cfblk1)
  cfblk322/1 -> cyemi_1733/1
  cyemi_1734/1 -> cfblk317/2(cfblk12)
  cfblk334/1 -> cyemi_1734/1
  cyemi_1735/1 -> cfblk317/3(cfblk13)
  cfblk209/1 -> cyemi_1735/1
  cyemi_1736/1 -> cfblk317/4(cfblk14)
  cfblk310/1(cfblk2) -> cyemi_1736/1
  cyemi_1737/1 -> cfblk317/5(cfblk15)
  cfblk358/1 -> cyemi_1737/1
  cyemi_1738/1 -> cfblk317/6(cfblk16)
  cfblk363/1 -> cyemi_1738/1
  cyemi_1768/1 -> cfblk318/1(cfblk1)
  cfblk269/1(cfblk2) -> cyemi_1768/1
  cyemi_1769/1 -> cfblk318/2(cfblk13)
  cfblk219/1 -> cyemi_1769/1
  cyemi_1813/1 -> cfblk319/1(cfblk1)
  cfblk289/2(cfblk9) -> cyemi_1813/1
  cyemi_1814/1 -> cfblk319/2(cfblk11)
  cfblk366/1 -> cyemi_1814/1
  cyemi_1815/1 -> cfblk319/3(cfblk12)
  cyemi_1816/1 -> cfblk319/4(cfblk13)
  cfblk354/1 -> cyemi_1816/1
  cyemi_1817/1 -> cfblk319/5(cfblk14)
  cyemi_1829/1 -> cfblk32/1
  cyemi_1830/1 -> cfblk320/1
  cfblk297/1(cfblk2) -> cyemi_1830/1
  cyemi_1831/1 -> cfblk321/1
  cfblk27/1 -> cyemi_1831/1
  cyemi_1832/1 -> cfblk322/1
  cfblk20/1 -> cyemi_1832/1
  cyemi_1833/1 -> cfblk323/1
  cfblk26/1 -> cyemi_1833/1
  cyemi_1834/1 -> cfblk324/1
  cfblk82/1 -> cyemi_1834/1
  cyemi_1835/1 -> cfblk325/1
  cfblk61/1 -> cyemi_1835/1
  cyemi_1836/1 -> cfblk326/1
  cfblk284/2(cfblk12) -> cyemi_1836/1
  cyemi_1837/1 -> cfblk327/1
  cfblk3/1 -> cyemi_1837/1
  cyemi_1838/1 -> cfblk328/1
  cyemi_1839/1 -> cfblk329/1
  cyemi_1840/1 -> cfblk33/1
  cyemi_1841/1 -> cfblk330/1
  cfblk276/2(cfblk12) -> cyemi_1841/1
  cyemi_1842/1 -> cfblk331/1
  cyemi_1843/1 -> cfblk332/1
  cyemi_1844/1 -> cfblk333/1
  cyemi_1845/1 -> cfblk334/1
  cyemi_1846/1 -> cfblk335/1
  cyemi_1847/1 -> cfblk336/1
  cfblk298/1(cfblk2) -> cyemi_1847/1
  cyemi_1848/1 -> cfblk337/1
  cyemi_1849/1 -> cfblk338/1
  cyemi_1850/1 -> cfblk339/1
  cfblk9/1 -> cyemi_1850/1
  cyemi_1851/1 -> cfblk34/1
  cfblk273/1(cfblk2) -> cyemi_1851/1
  cyemi_1852/1 -> cfblk340/1
  cyemi_1853/1 -> cfblk341/1
  cfblk288/3(cfblk13) -> cyemi_1853/1
  cyemi_1854/1 -> cfblk342/1
  cyemi_1855/1 -> cfblk343/1
  cfblk29/1 -> cyemi_1855/1
  cyemi_1856/1 -> cfblk344/1
  cfblk36/1 -> cyemi_1856/1
  cyemi_1857/1 -> cfblk345/1
  cfblk258/3(cfblk17) -> cyemi_1857/1
  cyemi_1858/1 -> cfblk346/1
  cfblk6/1 -> cyemi_1858/1
  cyemi_1859/1 -> cfblk347/1
  cfblk271/2(cfblk14) -> cyemi_1859/1
  cyemi_1860/1 -> cfblk348/1
  cfblk311/2(cfblk15) -> cyemi_1860/1
  cyemi_1861/1 -> cfblk349/1
  cfblk272/1(cfblk2) -> cyemi_1861/1
  cyemi_1862/1 -> cfblk35/1
  cfblk302/2(cfblk8) -> cyemi_1862/1
  cyemi_1863/1 -> cfblk350/1
  cyemi_1864/1 -> cfblk351/1
  cfblk97/1 -> cyemi_1864/1
  cyemi_1865/1 -> cfblk352/1
  cyemi_1866/1 -> cfblk353/1
  cyemi_1867/1 -> cfblk354/1
  cyemi_1868/1 -> cfblk355/1
  cfblk302/1(cfblk2) -> cyemi_1868/1
  cyemi_1869/1 -> cfblk356/1
  cfblk106/1 -> cyemi_1869/1
  cyemi_1870/1 -> cfblk357/1
  cfblk91/1 -> cyemi_1870/1
  cyemi_1871/1 -> cfblk358/1
  cfblk261/2(cfblk13) -> cyemi_1871/1
  cyemi_1872/1 -> cfblk359/1
  cfblk281/1(cfblk2) -> cyemi_1872/1
  cyemi_1873/1 -> cfblk36/1
  cfblk294/1(cfblk2) -> cyemi_1873/1
  cyemi_1874/1 -> cfblk360/1
  cfblk281/2(cfblk7) -> cyemi_1874/1
  cyemi_1875/1 -> cfblk361/1
  cfblk291/1(cfblk2) -> cyemi_1875/1
  cyemi_1876/1 -> cfblk362/1
  cfblk66/1 -> cyemi_1876/1
  cyemi_1877/1 -> cfblk363/1
  cfblk283/3(cfblk8) -> cyemi_1877/1
  cyemi_1878/1 -> cfblk364/1
  cyemi_1879/1 -> cfblk365/1
  cfblk291/3(cfblk13) -> cyemi_1879/1
  cyemi_1880/1 -> cfblk366/1
  cyemi_1881/1 -> cfblk367/1
  cfblk76/1 -> cyemi_1881/1
  cyemi_1882/1 -> cfblk368/1
  cfblk70/1 -> cyemi_1882/1
  cyemi_1883/1 -> cfblk369/1
  cfblk301/2(cfblk16) -> cyemi_1883/1
  cyemi_1884/1 -> cfblk37/1
  cfblk202/1 -> cyemi_1884/1
  cyemi_1885/1 -> cfblk370/1
  cfblk297/2(cfblk12) -> cyemi_1885/1
  cyemi_1886/1 -> cfblk371/1
  cfblk318/3(cfblk15) -> cyemi_1886/1
  cyemi_1887/1 -> cfblk372/1
  cfblk286/3(cfblk9) -> cyemi_1887/1
  cyemi_1888/1 -> cfblk373/1
  cfblk267/2(cfblk17) -> cyemi_1888/1
  cyemi_1889/1 -> cfblk374/1
  cfblk40/1 -> cyemi_1889/1
  cyemi_1890/1 -> cfblk375/1
  cyemi_1891/1 -> cfblk376/1
  cfblk110/1 -> cyemi_1891/1
  cyemi_1892/1 -> cfblk377/1
  cfblk174/1 -> cyemi_1892/1
  cyemi_1893/1 -> cfblk378/1
  cfblk57/1 -> cyemi_1893/1
  cyemi_1894/1 -> cfblk379/1
  cfblk216/1 -> cyemi_1894/1
  cyemi_1895/1 -> cfblk38/1
  cyemi_1896/1 -> cfblk39/1
  cfblk286/1(cfblk2) -> cyemi_1896/1
  cyemi_1897/1 -> cfblk4/1
  cfblk17/1 -> cyemi_1897/1
  cyemi_1898/1 -> cfblk40/1
  cyemi_1899/1 -> cfblk41/1
  cfblk259/2(cfblk14) -> cyemi_1899/1
  cyemi_1900/1 -> cfblk42/1
  cyemi_1901/1 -> cfblk43/1
  cyemi_1902/1 -> cfblk44/1
  cfblk205/1 -> cyemi_1902/1
  cyemi_1903/1 -> cfblk45/1
  cfblk173/1 -> cyemi_1903/1
  cyemi_1904/1 -> cfblk46/1
  cfblk102/1 -> cyemi_1904/1
  cyemi_1905/1 -> cfblk47/1
  cyemi_1906/1 -> cfblk48/1
  cfblk105/1 -> cyemi_1906/1
  cyemi_1907/1 -> cfblk48/2
  cfblk305/2(cfblk11) -> cyemi_1907/1
  cyemi_1908/1 -> cfblk49/1
  cfblk307/1(cfblk2) -> cyemi_1908/1
  cyemi_1909/1 -> cfblk5/1
  cyemi_1910/1 -> cfblk50/1
  cfblk203/1 -> cyemi_1910/1
  cyemi_1911/1 -> cfblk51/1
  cfblk225/1 -> cyemi_1911/1
  cyemi_1912/1 -> cfblk52/1
  cfblk217/1 -> cyemi_1912/1
  cyemi_1913/1 -> cfblk53/1
  cfblk223/1 -> cyemi_1913/1
  cyemi_1914/1 -> cfblk54/1
  cfblk287/3(cfblk14) -> cyemi_1914/1
  cyemi_1915/1 -> cfblk55/1
  cfblk214/1(Signal 1) -> cyemi_1915/1
  cyemi_1916/1 -> cfblk56/1
  cyemi_1917/1 -> cfblk57/1
  cfblk379/1 -> cyemi_1917/1
  cyemi_1918/1 -> cfblk58/1
  cfblk101/1 -> cyemi_1918/1
  cyemi_1919/1 -> cfblk59/1
  cfblk296/1(cfblk2) -> cyemi_1919/1
  cyemi_1920/1 -> cfblk6/1
  cfblk73/1 -> cyemi_1920/1
  cyemi_1921/1 -> cfblk60/1
  cfblk264/2(cfblk14) -> cyemi_1921/1
  cyemi_1922/1 -> cfblk61/1
  cyemi_1923/1 -> cfblk62/1
  cfblk95/1 -> cyemi_1923/1
  cyemi_1924/1 -> cfblk63/1
  cfblk288/2(cfblk12) -> cyemi_1924/1
  cyemi_1925/1 -> cfblk64/1
  cfblk54/1 -> cyemi_1925/1
  cyemi_1926/1 -> cfblk65/1
  cfblk263/1(cfblk2) -> cyemi_1926/1
  cyemi_1927/1 -> cfblk66/1
  cyemi_1928/1 -> cfblk66/2
  cyemi_1929/1 -> cfblk67/1
  cfblk318/2(cfblk14) -> cyemi_1929/1
  cyemi_1930/1 -> cfblk68/1
  cfblk298/2(cfblk13) -> cyemi_1930/1
  cyemi_1931/1 -> cfblk69/1
  cfblk72/1 -> cyemi_1931/1
  cyemi_1932/1 -> cfblk7/1
  cfblk287/1(cfblk2) -> cyemi_1932/1
  cyemi_1933/1 -> cfblk70/1
  cyemi_1934/1 -> cfblk71/1
  cfblk189/1 -> cyemi_1934/1
  cyemi_1935/1 -> cfblk71/2
  cfblk317/1(cfblk2) -> cyemi_1935/1
  cyemi_1936/1 -> cfblk72/1
  cfblk2/1 -> cyemi_1936/1
  cyemi_1937/1 -> cfblk72/2
  cfblk258/2(cfblk16) -> cyemi_1937/1
  cyemi_1938/1 -> cfblk73/1
  cfblk109/1 -> cyemi_1938/1
  cyemi_1939/1 -> cfblk73/2
  cfblk211/1 -> cyemi_1939/1
  cyemi_1940/1 -> cfblk74/1
  cfblk33/1 -> cyemi_1940/1
  cyemi_1941/1 -> cfblk74/2
  cfblk88/1 -> cyemi_1941/1
  cyemi_1942/1 -> cfblk75/1
  cfblk21/1 -> cyemi_1942/1
  cyemi_1943/1 -> cfblk76/1
  cyemi_1944/1 -> cfblk77/1
  cfblk314/1(cfblk2) -> cyemi_1944/1
  cyemi_1945/1 -> cfblk78/1
  cyemi_1946/1 -> cfblk78/2
  cyemi_1947/1 -> cfblk79/1
  cfblk269/4(cfblk17) -> cyemi_1947/1
  cyemi_1948/1 -> cfblk8/1
  cfblk23/1 -> cyemi_1948/1
  cyemi_1949/1 -> cfblk80/1
  cfblk315/1(cfblk2) -> cyemi_1949/1
  cyemi_1950/1 -> cfblk80/2
  cfblk320/1 -> cyemi_1950/1
  cyemi_1951/1 -> cfblk81/1
  cyemi_1952/1 -> cfblk82/1
  cfblk259/1(cfblk2) -> cyemi_1952/1
  cyemi_1953/1 -> cfblk83/1
  cfblk187/1 -> cyemi_1953/1
  cyemi_1954/1 -> cfblk84/1
  cfblk295/1(cfblk2) -> cyemi_1954/1
  cyemi_1955/1 -> cfblk85/1
  cfblk5/1 -> cyemi_1955/1
  cyemi_1956/1 -> cfblk86/1
  cfblk190/1 -> cyemi_1956/1
  cyemi_1957/1 -> cfblk87/1
  cyemi_1958/1 -> cfblk87/2
  cfblk291/2(cfblk12) -> cyemi_1958/1
  cyemi_1959/1 -> cfblk88/1
  cfblk265/3(cfblk10) -> cyemi_1959/1
  cyemi_1960/1 -> cfblk89/1
  cfblk14/1 -> cyemi_1960/1
  cyemi_1961/1 -> cfblk9/1
  cfblk104/1 -> cyemi_1961/1
  cyemi_1962/1 -> cfblk90/1
  cfblk279/2(cfblk8) -> cyemi_1962/1
  cyemi_1963/1 -> cfblk91/1
  cfblk19/1 -> cyemi_1963/1
  cyemi_1964/1 -> cfblk92/1
  cfblk261/3(cfblk14) -> cyemi_1964/1
  cyemi_1965/1 -> cfblk92/2
  cyemi_1966/1 -> cfblk93/1
  cfblk100/1 -> cyemi_1966/1
  cyemi_1967/1 -> cfblk93/2
  cyemi_1968/1 -> cfblk94/1
  cfblk200/1(Signal 1) -> cyemi_1968/1
  cyemi_1969/1 -> cfblk95/1
  cfblk69/1 -> cyemi_1969/1
  cyemi_1970/1 -> cfblk96/1
  cfblk261/4(cfblk15) -> cyemi_1970/1
  cyemi_1971/1 -> cfblk97/1
  cfblk50/1 -> cyemi_1971/1
  cyemi_1972/1 -> cfblk97/2
  cfblk285/2(cfblk13) -> cyemi_1972/1
  cyemi_1973/1 -> cfblk98/1
  cfblk260/2(cfblk15) -> cyemi_1973/1
  cyemi_1974/1 -> cfblk99/1
  cfblk378/1 -> cyemi_1974/1

== system sampleModel7288_pp_1_1/cfblk200 ==
  Demux : Demux  Tag=STV Demux  Outputs=1
  FromWs : FromWorkspace  Tag=STV FromWs  VariableName=tuvar  SampleTime=0
      SigBuilderData=|
      | common.afterFinalStr = 'Extrapolate'
      | common.sampleTime = 0
      | dataSet.timeRange = [0 10]
      | dataSet.name = 'Group 1'
      | sbobj.Groups.Name = 'Group 1'
      | sbobj.Groups.Signals.Name = 'Signal 1'
      | sbobj.Groups.Signals.XData = [0 4 4 6 6 10]
      | sbobj.Groups.Signals.YData = [0 0 1 1 0 0]
  Signal 1 : Outport  Tag=STV Outport
  wires:
  Demux/1 -> Signal 1/1
  FromWs/1 -> Demux/1

== system sampleModel7288_pp_1_1/cfblk214 ==
  Demux : Demux  Tag=STV Demux  Outputs=1
  FromWs : FromWorkspace  Tag=STV FromWs  VariableName=tuvar  SampleTime=0
      SigBuilderData=|
      | common.afterFinalStr = 'Extrapolate'
      | common.sampleTime = 0
      | dataSet.timeRange = [0 10]
      | dataSet.name = 'Group 1'
      | sbobj.Groups.Name = 'Group 1'
      | sbobj.Groups.Signals.Name = 'Signal 1'
      | sbobj.Groups.Signals.XData = [0 4 4 6 6 10]
      | sbobj.Groups.Signals.YData = [0 0 1 1 0 0]
  Signal 1 : Outport  Tag=STV Outport
  wires:
  Demux/1 -> Signal 1/1
  FromWs/1 -> Demux/1

== system sampleModel7288_pp_1_1/cfblk215 ==
  Demux : Demux  Tag=STV Demux  Outputs=1
  FromWs : FromWorkspace  Tag=STV FromWs  VariableName=tuvar  SampleTime=0
      SigBuilderData=|
      | common.afterFinalStr = 'Extrapolate'
      | common.sampleTime = 0
      | dataSet.timeRange = [0 10]
      | dataSet.name = 'Group 1'
      | sbobj.Groups.Name = 'Group 1'
      | sbobj.Groups.Signals.Name = 'Signal 1'
      | sbobj.Groups.Signals.XData = [0 4 4 6 6 10]
      | sbobj.Groups.Signals.YData = [0 0 1 1 0 0]
  Signal 1 : Outport  Tag=STV Outport
  wires:
  Demux/1 -> Signal 1/1
  FromWs/1 -> Demux/1

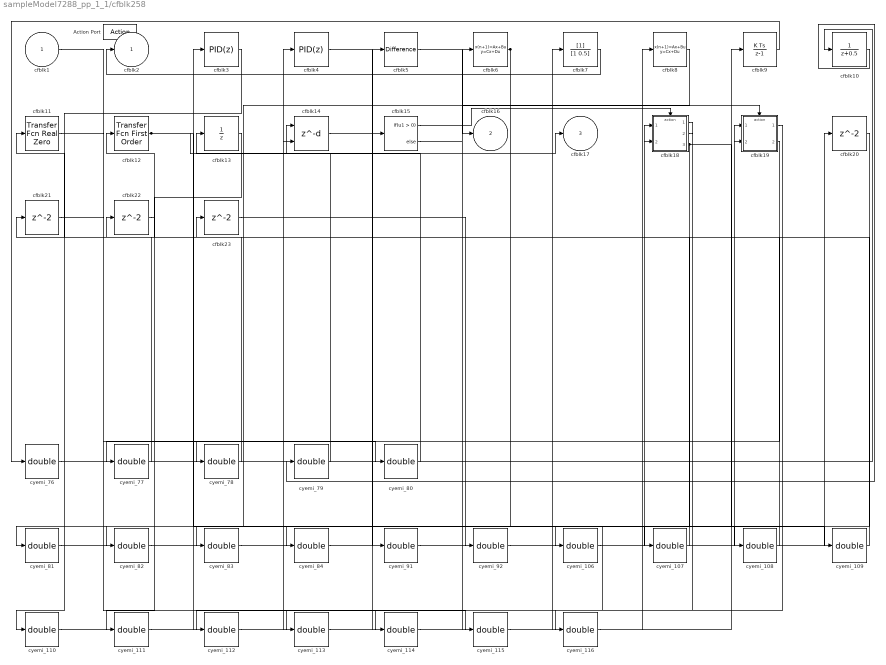
== system sampleModel7288_pp_1_1/cfblk258 ==
  cfblk1 : Inport
  Action Port : ActionPort  ActionType=then
  cfblk10 : DiscreteTransferFcn
  cfblk11 : simulink/Discrete/Transfer Fcn Real Zero  ZeroZ=0.75  ICPrevInput=0.0  DoSatur=off
      settings: SourceProductName=Simulink  SourceProductBaseCode=SL
  cfblk12 : simulink/Discrete/Transfer Fcn First Order  PoleZ=0.95  ICPrevOutput=0.0  DoSatur=off
      settings: SourceProductName=Simulink
  cfblk13 : UnitDelay  SampleTime=-1
  cfblk14 : Delay  DelayLengthSource=Input port
      settings: InputPortMap=u0,p1
  cfblk15 : If  SampleTime=1
  cfblk18 : Subsystem  TreatAsAtomicUnit=on
  cfblk19 : Subsystem  TreatAsAtomicUnit=on
  cfblk{20..23} (4 alike) : Delay
  cfblk3 : simulink/Continuous/PID Controller  Controller=PID  TimeDomain=Discrete-time  SampleTime=-1  IntegratorMethod=Forward Euler  FilterMethod=Forward Euler  Form=Parallel  UseFilter=on  ControllerParametersSource=internal  P=1  I=1  D=0  N=100  InitialConditionSource=internal  InitialConditionForIntegrator=0  InitialConditionForFilter=0  ExternalReset=none  LimitOutput=off  UpperSaturationLimit=inf  LowerSaturationLimit=-inf  LinearizeAsGain=off  AntiWindupMode=none  Kb=1  TrackingMode=off  Kt=1  PParamMin=[]  PParamMax=[]  IParamMin=[]  IParamMax=[]  DParamMin=[]  DParamMax=[]  NParamMin=[]  NParamMax=[]  KbParamMin=[]  KbParamMax=[]  KtParamMin=[]  KtParamMax=[]  POutMin=[]  POutMax=[]  IOutMin=[]  IOutMax=[]  DOutMin=[]  DOutMax=[]  NOutMin=[]  NOutMax=[]  KbOutMin=[]  KbOutMax=[]  KtOutMin=[]  KtOutMax=[]  IntegratorOutMin=[]  IntegratorOutMax=[]  FilterOutMin=[]  FilterOutMax=[]  SumOutMin=[]  SumOutMax=[]  SumI1OutMin=[]  SumI1OutMax=[]  SumI2OutMin=[]  SumI2OutMax=[]  SumI3OutMin=[]  SumI3OutMax=[]  SumDOutMin=[]  SumDOutMax=[]  SaturationOutMin=[]  SaturationOutMax=[]  IntegratorContinuousStateAttributes=''  IntegratorStateMustResolveToSignalObject=off  IntegratorRTWStateStorageClass=Auto  FilterContinuousStateAttributes=''  FilterStateMustResolveToSignalObject=off  FilterRTWStateStorageClass=Auto  DifferentiatorICPrevScaledInput=0  DifferentiatorOutMin=[]  DifferentiatorOutMax=[]  FilterDiffOutCoefMin=[]  FilterDiffOutCoefMax=[]  SumDenOutMin=[]  SumDenOutMax=[]  SumNumOutMin=[]  SumNumOutMax=[]  ReciprocalOutMin=[]  ReciprocalOutMax=[]  DivideOutMin=[]  DivideOutMax=[]  TunerSelectOption=Transfer Function Based (PID Tuner App)
  cfblk4 : simulink/Continuous/PID Controller  Controller=PID  TimeDomain=Discrete-time  SampleTime=-1  IntegratorMethod=Forward Euler  FilterMethod=Forward Euler  Form=Parallel  UseFilter=on  ControllerParametersSource=internal  P=1  I=1  D=0  N=100  InitialConditionSource=internal  InitialConditionForIntegrator=0  InitialConditionForFilter=0  ExternalReset=none  LimitOutput=off  UpperSaturationLimit=inf  LowerSaturationLimit=-inf  LinearizeAsGain=off  AntiWindupMode=none  Kb=1  TrackingMode=off  Kt=1  PParamMin=[]  PParamMax=[]  IParamMin=[]  IParamMax=[]  DParamMin=[]  DParamMax=[]  NParamMin=[]  NParamMax=[]  KbParamMin=[]  KbParamMax=[]  KtParamMin=[]  KtParamMax=[]  POutMin=[]  POutMax=[]  IOutMin=[]  IOutMax=[]  DOutMin=[]  DOutMax=[]  NOutMin=[]  NOutMax=[]  KbOutMin=[]  KbOutMax=[]  KtOutMin=[]  KtOutMax=[]  IntegratorOutMin=[]  IntegratorOutMax=[]  FilterOutMin=[]  FilterOutMax=[]  SumOutMin=[]  SumOutMax=[]  SumI1OutMin=[]  SumI1OutMax=[]  SumI2OutMin=[]  SumI2OutMax=[]  SumI3OutMin=[]  SumI3OutMax=[]  SumDOutMin=[]  SumDOutMax=[]  SaturationOutMin=[]  SaturationOutMax=[]  IntegratorContinuousStateAttributes=''  IntegratorStateMustResolveToSignalObject=off  IntegratorRTWStateStorageClass=Auto  FilterContinuousStateAttributes=''  FilterStateMustResolveToSignalObject=off  FilterRTWStateStorageClass=Auto  DifferentiatorICPrevScaledInput=0  DifferentiatorOutMin=[]  DifferentiatorOutMax=[]  FilterDiffOutCoefMin=[]  FilterDiffOutCoefMax=[]  SumDenOutMin=[]  SumDenOutMax=[]  SumNumOutMin=[]  SumNumOutMax=[]  ReciprocalOutMin=[]  ReciprocalOutMax=[]  DivideOutMin=[]  DivideOutMax=[]  TunerSelectOption=Transfer Function Based (PID Tuner App)
  cfblk5 : simulink/Discrete/Difference  ICPrevInput=0.0  OutMin=[]  OutMax=[]  OutDataTypeStr=double  OutputDataTypeScalingMode=double  OutDataType=fixdt(1, 16)  OutScaling=2^-10  DoSatur=off
  cfblk6 : DiscreteStateSpace  SampleTime=-1
  cfblk7 : DiscreteFilter
  cfblk8 : DiscreteStateSpace  SampleTime=-1
  cfblk9 : DiscreteIntegrator  SampleTime=-1  OutDataTypeStr=double  ICPrevOutput=DiscIntNeverNeededParam  ICPrevScaledInput=DiscIntNeverNeededParam
  cyemi_{76..84,91..92,106..116} (22 alike) : DataTypeConversion  OutDataTypeStr=double
  cfblk2 : Outport
  cfblk16 : Outport  Port=2
  cfblk17 : Outport  Port=3
  wires:
  cfblk7/1 -> cfblk2/1
  cfblk12/1 -> cfblk17/1, cyemi_106/1
  cfblk5/1 -> cfblk16/1
  cfblk18/3(cfblk9) -> cyemi_109/1, cyemi_116/1
  cfblk6/1 -> cyemi_77/1, cyemi_110/1
  cfblk15/1 -> cfblk18/Action
  cfblk15/2 -> cfblk19/Action
  cyemi_76/1 -> cfblk10/1
  cfblk9/1 -> cyemi_76/1
  cyemi_77/1 -> cfblk11/1
  cyemi_78/1 -> cfblk12/1
  cfblk19/2(cfblk16) -> cyemi_78/1
  cyemi_79/1 -> cfblk13/1
  cfblk10/1 -> cyemi_79/1
  cyemi_80/1 -> cfblk14/1
  cfblk21/1 -> cyemi_80/1
  cyemi_81/1 -> cfblk14/2
  cfblk3/1 -> cyemi_81/1
  cyemi_82/1 -> cfblk15/1
  cfblk22/1 -> cyemi_82/1
  cyemi_83/1 -> cfblk18/1(cfblk1)
  cfblk8/1 -> cyemi_83/1
  cyemi_84/1 -> cfblk18/2(cfblk7)
  cfblk20/1 -> cyemi_84/1
  cyemi_91/1 -> cfblk19/1(cfblk1)
  cfblk14/1 -> cyemi_91/1
  cyemi_92/1 -> cfblk19/2(cfblk15)
  cfblk23/1 -> cyemi_92/1
  cyemi_106/1 -> cfblk20/1
  cyemi_107/1 -> cfblk21/1
  cfblk18/2(cfblk8) -> cyemi_107/1
  cyemi_108/1 -> cfblk22/1
  cfblk4/1 -> cyemi_108/1
  cyemi_109/1 -> cfblk23/1
  cyemi_110/1 -> cfblk3/1
  cyemi_111/1 -> cfblk4/1
  cfblk13/1 -> cyemi_111/1
  cyemi_112/1 -> cfblk5/1
  cfblk18/1(cfblk2) -> cyemi_112/1
  cyemi_113/1 -> cfblk6/1
  cfblk1/1 -> cyemi_113/1
  cyemi_114/1 -> cfblk7/1
  cfblk19/1(cfblk2) -> cyemi_114/1
  cyemi_115/1 -> cfblk8/1
  cfblk11/1 -> cyemi_115/1
  cyemi_116/1 -> cfblk9/1
